simulink model "model2"  (R2022a)
settings: Solver=VariableStepAuto  StartTime=0.0  StopTime=10.0  RelTol=1e-3
libraries: simulink_extras x1
settings Model: Creator=Ekaterina  LastModifiedBy=Ekaterina

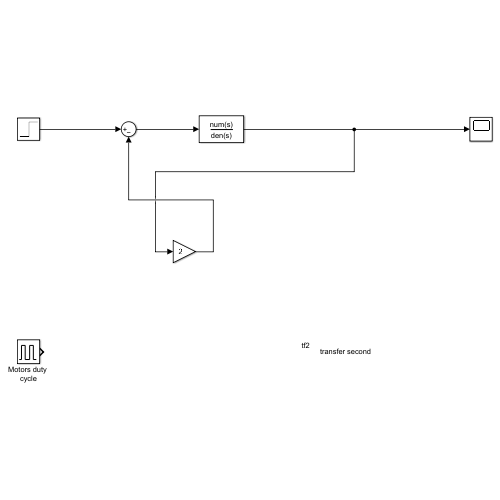
[thumbnail: Simulink's stored preview of the top-level diagram]
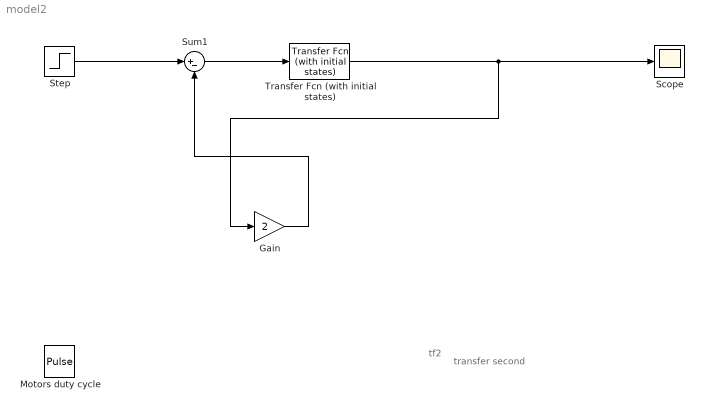
== system model2 ==
  note: transfer second
  note: tf2
  Gain : Gain  Gain=2
  Motors duty cycle : DiscretePulseGenerator  PulseType=Time based  Period=10  PulseWidth=40
  Scope : Scope
  Step : Step  Time=0.1  SampleTime=100
  Sum1 : Sum  Inputs=|+-
  Transfer Fcn (with initial states) : simulink_extras/Additional Linear/Transfer Fcn (with initial states)  N=[0 0 8.914 5.959 ]  D="[1  0.4083 1.017 0.1075]"  X0=.01
  wires:
  Gain/1 -> Sum1/2
  Transfer Fcn (with initial states)/1 -> Gain/1, Scope/1
  Step/1 -> Sum1/1
  Sum1/1 -> Transfer Fcn (with initial states)/1
